simulink model "PIDController"  (R2025a)
settings: Solver=VariableStepAuto  StartTime=0.0  StopTime=10.0  RelTol=1e-3
undefined symbols (not defined in the file): Kd, Ki, Kp
settings Model: Creator=Pablo  LastModifiedBy=Pablo

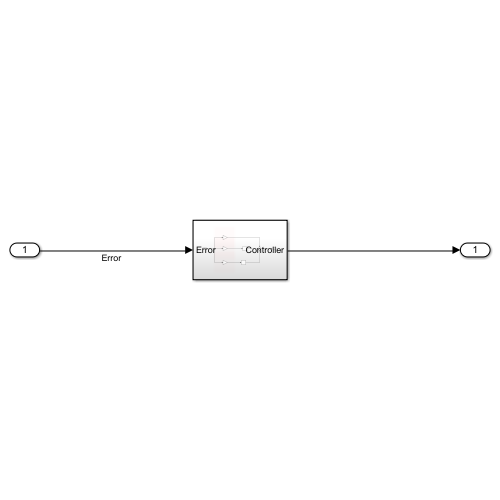
[thumbnail: Simulink's stored preview of the top-level diagram]
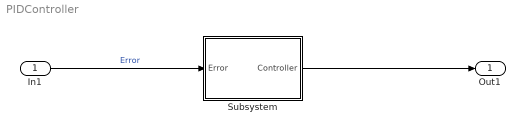
== system PIDController ==
  In1 : Inport
  Subsystem : Subsystem
  Out1 : Outport
  wires:
  In1/1 -> Subsystem/1(Error)  "Error"
  Subsystem/1(Controller) -> Out1/1

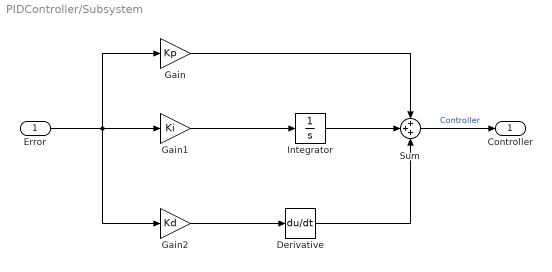
== system PIDController/Subsystem ==
  Error : Inport
  Derivative : Derivative
  Gain : Gain  Gain=Kp
  Gain1 : Gain  Gain=Ki
  Gain2 : Gain  Gain=Kd
  Integrator : Integrator
  Sum : Sum  Inputs=+++
  Controller : Outport
  wires:
  Sum/1 -> Controller/1  "Controller"
  Derivative/1 -> Sum/3
  Integrator/1 -> Sum/2
  Gain1/1 -> Integrator/1
  Gain/1 -> Sum/1
  Error/1 -> Gain2/1, Gain/1, Gain1/1
  Gain2/1 -> Derivative/1
